simulink model "IEEE30_case"  (R2024b)
settings: Solver=FixedStepAuto  StartTime=0  StopTime=5  FixedStep=1e-7  RelTol=1e-3
values from neighbouring files (symbols this model uses):
  GFL_DFIG_7_C_bus = 0.08    [IEEE30_case_parameters.m]
  GFL_DFIG_7_D_mutual = 2.500000e+3    (= 2500)    [IEEE30_case_parameters.m]
  GFL_DFIG_7_f0 = 60    [IEEE30_case_parameters.m]
  GFL_DFIG_7_gPLLi = 3200    [IEEE30_case_parameters.m]
  GFL_DFIG_7_gPLLp = 650    [IEEE30_case_parameters.m]
  GFL_DFIG_7_H_WT = 0.4    [IEEE30_case_parameters.m]
  GFL_DFIG_7_Hg = 0.8    [IEEE30_case_parameters.m]
  GFL_DFIG_7_Igq_ref = 0    [IEEE30_case_parameters.m]
  GFL_DFIG_7_Ird_ref = 704.45696    [IEEE30_case_parameters.m]
  GFL_DFIG_7_KI_V = -300000    [IEEE30_case_parameters.m]
  GFL_DFIG_7_KP_V = -1000    [IEEE30_case_parameters.m]
  GFL_DFIG_7_Ksh = 1.254300e+4    (= 12543)    [IEEE30_case_parameters.m]
  GFL_DFIG_7_Lg = 0.000483    [IEEE30_case_parameters.m]
  GFL_DFIG_7_Lm_pu = 4    [IEEE30_case_parameters.m]
  GFL_DFIG_7_N = 100    [IEEE30_case_parameters.m]
  GFL_DFIG_7_p = 2    [IEEE30_case_parameters.m]
  GFL_DFIG_7_Pitch = 0    [IEEE30_case_parameters.m]
  GFL_DFIG_7_R = 44    [IEEE30_case_parameters.m]
  GFL_DFIG_7_Rg = 2.000000e-5    (= 2e-05)    [IEEE30_case_parameters.m]
  GFL_DFIG_7_rho = 1.225    [IEEE30_case_parameters.m]
  GFL_DFIG_7_rPLLi = 4500    [IEEE30_case_parameters.m]
  GFL_DFIG_7_rPLLp = 620    [IEEE30_case_parameters.m]
  GFL_DFIG_7_Rs_pu = 0.011    [IEEE30_case_parameters.m]
  GFL_DFIG_7_Sbase = 2.000000e+6    (= 2000000)    [IEEE30_case_parameters.m]
  GFL_DFIG_7_ugq_ref = 0    [IEEE30_case_parameters.m]
  GFL_DFIG_7_usd_ref = 0    [IEEE30_case_parameters.m]
  GFL_DFIG_7_Vbase = 690    [IEEE30_case_parameters.m]
  GFL_DFIG_7_Vdc_ref = 1200    [IEEE30_case_parameters.m]
  GFL_DFIG_7_wind = 12    [IEEE30_case_parameters.m]
  GFL_DFIG_7_wm_ref = 518.184209    [IEEE30_case_parameters.m]
  SG_D_13_D = 0.01056    [IEEE30_case_parameters.m]
  SG_D_13_EnableSaturation = 0    [IEEE30_case_parameters.m]
  SG_D_13_f0 = 60    [IEEE30_case_parameters.m]
  SG_D_13_H = 7.5    [IEEE30_case_parameters.m]
  SG_D_13_K_A = 20    [IEEE30_case_parameters.m]
  SG_D_13_K_E = 1.000000e+1    (= 10)    [IEEE30_case_parameters.m]
  SG_D_13_K_F = 2.363    [IEEE30_case_parameters.m]
  SG_D_13_K_s = 0.5    [IEEE30_case_parameters.m]
  SG_D_13_R_a = 0.001088    [IEEE30_case_parameters.m]
  SG_D_13_S_A = 1    [IEEE30_case_parameters.m]
  SG_D_13_S_B = 0.103    [IEEE30_case_parameters.m]
  SG_D_13_S_N = 10.659857    [IEEE30_case_parameters.m]
  SG_D_13_SpeedPara = 200    [IEEE30_case_parameters.m]
  SG_D_13_T_0 = 0.370163    [IEEE30_case_parameters.m]
  SG_D_13_T_1 = 0.3    [IEEE30_case_parameters.m]
  SG_D_13_T_2 = 0.05    [IEEE30_case_parameters.m]
  SG_D_13_T_3 = 0.02    [IEEE30_case_parameters.m]
  SG_D_13_T_4 = 0.005    [IEEE30_case_parameters.m]
  SG_D_13_T_A = 0.02    [IEEE30_case_parameters.m]
  SG_D_13_T_dd = 8.000000e+0    (= 8)    [IEEE30_case_parameters.m]
  SG_D_13_T_ddd = 0.04    [IEEE30_case_parameters.m]
  SG_D_13_T_E = 0.314    [IEEE30_case_parameters.m]
  SG_D_13_T_F = 0.35    [IEEE30_case_parameters.m]
  SG_D_13_T_qd = 0.8    [IEEE30_case_parameters.m]
  SG_D_13_T_qdd = 0.02    [IEEE30_case_parameters.m]
  SG_D_13_T_speed = 0.1    [IEEE30_case_parameters.m]
  SG_D_13_T_w = 0.5    [IEEE30_case_parameters.m]
  SG_D_13_V_ref = 1.696619    [IEEE30_case_parameters.m]
  SG_D_13_w_ref = 376.991118    [IEEE30_case_parameters.m]
  SG_D_13_x_d = 1.9    [IEEE30_case_parameters.m]
  SG_D_13_x_dd = 0.302    [IEEE30_case_parameters.m]
  SG_D_13_x_ddd = 0.204    [IEEE30_case_parameters.m]
  SG_D_13_x_l = 0.05    [IEEE30_case_parameters.m]
  SG_D_13_x_q = 1.3    [IEEE30_case_parameters.m]
  SG_D_13_x_qd = 0.5    [IEEE30_case_parameters.m]
  SG_D_13_x_qdd = 0.3    [IEEE30_case_parameters.m]
  SG_D_1_D = 0.01056    [IEEE30_case_parameters.m]
  SG_D_1_EnableSaturation = 0    [IEEE30_case_parameters.m]
  SG_D_1_f0 = 60    [IEEE30_case_parameters.m]
  SG_D_1_H = 7.5    [IEEE30_case_parameters.m]
  SG_D_1_K_A = 20    [IEEE30_case_parameters.m]
  SG_D_1_K_E = 1.000000e+1    (= 10)    [IEEE30_case_parameters.m]
  SG_D_1_K_F = 2.363    [IEEE30_case_parameters.m]
  SG_D_1_K_s = 0.5    [IEEE30_case_parameters.m]
  SG_D_1_R_a = 0.001088    [IEEE30_case_parameters.m]
  SG_D_1_S_A = 1    [IEEE30_case_parameters.m]
  SG_D_1_S_B = 0.103    [IEEE30_case_parameters.m]
  SG_D_1_S_N = 10.659857    [IEEE30_case_parameters.m]
  SG_D_1_SpeedPara = 200    [IEEE30_case_parameters.m]
  SG_D_1_T_0 = 0.259812    [IEEE30_case_parameters.m]
  SG_D_1_T_1 = 0.3    [IEEE30_case_parameters.m]
  SG_D_1_T_2 = 0.05    [IEEE30_case_parameters.m]
  SG_D_1_T_3 = 0.02    [IEEE30_case_parameters.m]
  SG_D_1_T_4 = 0.005    [IEEE30_case_parameters.m]
  SG_D_1_T_A = 0.02    [IEEE30_case_parameters.m]
  SG_D_1_T_dd = 8.000000e+0    (= 8)    [IEEE30_case_parameters.m]
  SG_D_1_T_ddd = 0.04    [IEEE30_case_parameters.m]
  SG_D_1_T_E = 0.314    [IEEE30_case_parameters.m]
  SG_D_1_T_F = 0.35    [IEEE30_case_parameters.m]
  SG_D_1_T_qd = 0.8    [IEEE30_case_parameters.m]
  SG_D_1_T_qdd = 0.02    [IEEE30_case_parameters.m]
  SG_D_1_T_speed = 0.1    [IEEE30_case_parameters.m]
  SG_D_1_T_w = 0.5    [IEEE30_case_parameters.m]
  SG_D_1_V_ref = 1.544107    [IEEE30_case_parameters.m]
  SG_D_1_w_ref = 376.991118    [IEEE30_case_parameters.m]
  SG_D_1_x_d = 1.9    [IEEE30_case_parameters.m]
  SG_D_1_x_dd = 0.302    [IEEE30_case_parameters.m]
  SG_D_1_x_ddd = 0.204    [IEEE30_case_parameters.m]
  SG_D_1_x_l = 0.05    [IEEE30_case_parameters.m]
  SG_D_1_x_q = 1.3    [IEEE30_case_parameters.m]
  SG_D_1_x_qd = 0.5    [IEEE30_case_parameters.m]
  SG_D_1_x_qdd = 0.3    [IEEE30_case_parameters.m]
  SG_D_22_D = 0.01056    [IEEE30_case_parameters.m]
  SG_D_22_EnableSaturation = 0    [IEEE30_case_parameters.m]
  SG_D_22_f0 = 60    [IEEE30_case_parameters.m]
  SG_D_22_H = 7.5    [IEEE30_case_parameters.m]
  SG_D_22_K_A = 20    [IEEE30_case_parameters.m]
  SG_D_22_K_E = 1.000000e+1    (= 10)    [IEEE30_case_parameters.m]
  SG_D_22_K_F = 2.363    [IEEE30_case_parameters.m]
  SG_D_22_K_s = 0.5    [IEEE30_case_parameters.m]
  SG_D_22_R_a = 0.001088    [IEEE30_case_parameters.m]
  SG_D_22_S_A = 1    [IEEE30_case_parameters.m]
  SG_D_22_S_B = 0.103    [IEEE30_case_parameters.m]
  SG_D_22_S_N = 10.659857    [IEEE30_case_parameters.m]
  SG_D_22_SpeedPara = 200    [IEEE30_case_parameters.m]
  SG_D_22_T_0 = 0.216121    [IEEE30_case_parameters.m]
  SG_D_22_T_1 = 0.3    [IEEE30_case_parameters.m]
  SG_D_22_T_2 = 0.05    [IEEE30_case_parameters.m]
  SG_D_22_T_3 = 0.02    [IEEE30_case_parameters.m]
  SG_D_22_T_4 = 0.005    [IEEE30_case_parameters.m]
  ... (+126 more)
(part 19 of 27)

== system IEEE30_case/SG_D_13/d_psi_q_SG_D_13_block ==
  note: d_psi_q_SG_D_13 in IEEE30_case
      | $2\,\pi \,f_{0}\,\left(v_{d,\mathrm{SG},D,13}\,\cos\left(\theta _{\mathrm{SG},D,13}\right)+v_{q,\mathrm{SG},D,13}\,\sin\left(\theta _{\mathrm{SG},D,13}\right)-\frac{R_{a}\,\left(\psi _{q,\mathrm{SG},D,13}+\frac{\psi _{\mathrm{gq},\mathrm{SG},D,13}\,\left(x_{l}-x_{\mathrm{qdd}}\right)}{x_{l}-x_{\mathrm{qd}}}+\frac{\psi _{\mathrm{kq},\mathrm{SG},D,13}\,\left(x_{\mathrm{qd}}-x_{\mathrm{qdd}}\right)}{x_{l}-x_{\mathrm{qd}}}\right)}{x_{\mathrm{qdd}}}-\frac{\psi _{d,\mathrm{SG},D,13}\,w_{\mathrm{SG},D,13}}{2\,f_{0}\,\pi }\right)$
      | Automatically generated on 2025-11-01 18:34:46 .
  State_psi_gq_SG_D_13_b9e70 : Inport
  State_psi_kq_SG_D_13_777e8 : Inport  Port=2
  State_psi_q_SG_D_13_352e5 : Inport  Port=3
  Input_v_d_SG_D_13_60103 : Inport  Port=4
  State_theta_SG_D_13_d73b7 : Inport  Port=5
  Input_v_q_SG_D_13_89396 : Inport  Port=6
  State_theta_SG_D_13_d24c4 : Inport  Port=7
  State_psi_d_SG_D_13_acca0 : Inport  Port=8
  State_w_SG_D_13_af3fa : Inport  Port=9
  Add_212ec : Sum
  Add_30131 : Sum
  Add_3345e : Sum
  Add_60563 : Sum
  Add_71f1c : Sum
  Constant_-1_23601 : Constant  Value=-1
  Constant_-1_802f8 : Constant  Value=-1
  Constant_-1_a74eb : Constant  Value=-1
  Constant_-2.0_d214a : Constant  Value=-2.0
  Constant_2.0_b6abe : Constant  Value=2.0
  Constant_R_a_2cc2b : Constant  Value=R_a
  Constant_f0_87ec9 : Constant  Value=f0
  Constant_f0_e30ed : Constant  Value=f0
  Constant_pi_494f1 : Constant  Value=pi
  Constant_pi_861ee : Constant  Value=pi
  Constant_x_l_134aa : Constant  Value=x_l
  Constant_x_l_cdd9f : Constant  Value=x_l
  Constant_x_l_e4e7e : Constant  Value=x_l
  Constant_x_qd_c3898 : Constant  Value=x_qd
  Constant_x_qd_e989e : Constant  Value=x_qd
  Constant_x_qd_f4ba2 : Constant  Value=x_qd
  Constant_x_qdd_25541 : Constant  Value=x_qdd
  Constant_x_qdd_713f8 : Constant  Value=x_qdd
  Constant_x_qdd_d4846 : Constant  Value=x_qdd
  Divide_26cb3 : Product  Inputs=*/
  Divide_92868 : Product  Inputs=*/
  Divide_950ba : Product  Inputs=*/
  Divide_db475 : Product  Inputs=*/
  MathFunc_cos_7503c : Trigonometry  Operator=cos
  MathFunc_sin_a8361 : Trigonometry
  Product_06178 : Product
  Product_316b1 : Product
  Product_3ac25 : Product
  Product_3c410 : Product
  Product_432cf : Product
  Product_5efb9 : Product
  Product_7509b : Product
  Product_9806d : Product
  Product_a5768 : Product
  Product_b8d96 : Product
  Product_ba2c3 : Product
  Product_bcc7a : Product
  Product_c3e4c : Product
  Product_de780 : Product
  Subtract_222ea : Sum  Inputs=+-
  Subtract_2db43 : Sum  Inputs=+-
  Subtract_b2b6c : Sum  Inputs=+-
  Subtract_cd486 : Sum  Inputs=+-
  Blockout_d_psi_q_SG_D_13_271e8 : Outport
  wires:
  Constant_f0_87ec9/1 -> Product_b8d96/2
  Constant_x_l_cdd9f/1 -> Product_316b1/2
  Constant_-1_802f8/1 -> Product_5efb9/1
  Product_5efb9/1 -> Add_212ec/1
  Subtract_222ea/1 -> Subtract_cd486/1
  Constant_x_l_e4e7e/1 -> Product_5efb9/2
  Subtract_b2b6c/1 -> Product_ba2c3/2
  Constant_x_qd_c3898/1 -> Subtract_b2b6c/1
  Constant_x_qdd_25541/1 -> Add_212ec/2
  Add_60563/1 -> Product_a5768/2
  Product_316b1/1 -> Add_71f1c/1
  Constant_-1_23601/1 -> Product_316b1/1
  Constant_-2.0_d214a/1 -> Product_432cf/1
  Constant_x_qdd_713f8/1 -> Subtract_b2b6c/2
  Constant_pi_861ee/1 -> Product_de780/2
  Product_a5768/1 -> Divide_92868/1
  Product_9806d/1 -> Add_30131/1
  Constant_-1_a74eb/1 -> Product_9806d/1
  Constant_x_l_134aa/1 -> Product_9806d/2
  Subtract_cd486/1 -> Add_3345e/1
  Product_c3e4c/1 -> Divide_950ba/1
  Constant_x_qd_e989e/1 -> Add_71f1c/2
  State_psi_gq_SG_D_13_b9e70/1 -> Product_c3e4c/1
  Add_212ec/1 -> Product_c3e4c/2
  Product_ba2c3/1 -> Divide_26cb3/1
  State_psi_kq_SG_D_13_777e8/1 -> Product_ba2c3/1
  Product_bcc7a/1 -> Divide_db475/2
  Constant_x_qd_f4ba2/1 -> Add_30131/2
  Add_71f1c/1 -> Divide_950ba/2
  Product_b8d96/1 -> Product_3ac25/1
  Add_30131/1 -> Divide_26cb3/2
  Divide_950ba/1 -> Subtract_2db43/1
  Subtract_2db43/1 -> Add_60563/1
  Divide_26cb3/1 -> Subtract_2db43/2
  State_psi_q_SG_D_13_352e5/1 -> Add_60563/2
  Product_3c410/1 -> Subtract_cd486/2
  Constant_R_a_2cc2b/1 -> Product_a5768/1
  State_theta_SG_D_13_d73b7/1 -> MathFunc_cos_7503c/1
  Constant_x_qdd_d4846/1 -> Divide_92868/2
  Product_7509b/1 -> Subtract_222ea/2
  Input_v_d_SG_D_13_60103/1 -> Product_7509b/1
  MathFunc_cos_7503c/1 -> Product_7509b/2
  Constant_f0_e30ed/1 -> Product_bcc7a/2
  MathFunc_sin_a8361/1 -> Product_3c410/2
  State_theta_SG_D_13_d24c4/1 -> MathFunc_sin_a8361/1
  Product_de780/1 -> Product_bcc7a/1
  Constant_2.0_b6abe/1 -> Product_de780/1
  Divide_92868/1 -> Subtract_222ea/1
  Input_v_q_SG_D_13_89396/1 -> Product_3c410/1
  Product_06178/1 -> Divide_db475/1
  State_psi_d_SG_D_13_acca0/1 -> Product_06178/1
  State_w_SG_D_13_af3fa/1 -> Product_06178/2
  Constant_pi_494f1/1 -> Product_432cf/2
  Divide_db475/1 -> Add_3345e/2
  Product_432cf/1 -> Product_b8d96/1
  Add_3345e/1 -> Product_3ac25/2
  Product_3ac25/1 -> Blockout_d_psi_q_SG_D_13_271e8/1

== system IEEE30_case/SG_D_13/d_theta_SG_D_13_block ==
  note: d_theta_SG_D_13 in IEEE30_case
      | $w_{\mathrm{SG},D,13}-2\,\pi \,f_{0}$
      | Automatically generated on 2025-11-01 18:35:09 .
  State_w_SG_D_13_8eb78 : Inport
  Add_5b0be : Sum
  Constant_-2.0_19a96 : Constant  Value=-2.0
  Constant_f0_3b1b7 : Constant  Value=f0
  Constant_pi_8ca32 : Constant  Value=pi
  Product_6dbd8 : Product
  Product_d020b : Product
  Blockout_d_theta_SG_D_13_8df5a : Outport
  wires:
  Constant_-2.0_19a96/1 -> Product_d020b/1
  Constant_pi_8ca32/1 -> Product_d020b/2
  Product_d020b/1 -> Product_6dbd8/1
  Constant_f0_3b1b7/1 -> Product_6dbd8/2
  Product_6dbd8/1 -> Add_5b0be/1
  State_w_SG_D_13_8eb78/1 -> Add_5b0be/2
  Add_5b0be/1 -> Blockout_d_theta_SG_D_13_8df5a/1

== system IEEE30_case/SG_D_13/d_w_SG_D_13_block ==
  note: d_w_SG_D_13 in IEEE30_case
      | $\frac{2\,\pi \,T_{m,\mathrm{SG},D,13}\,f_{0}-D\,\left(w_{\mathrm{SG},D,13}-2\,\pi \,f_{0}\right)+2\,\pi \,f_{0}\,\left(\frac{\psi _{d,\mathrm{SG},D,13}\,\left(\psi _{q,\mathrm{SG},D,13}+\frac{\psi _{\mathrm{gq},\mathrm{SG},D,13}\,\left(x_{l}-x_{\mathrm{qdd}}\right)}{x_{l}-x_{\mathrm{qd}}}+\frac{\psi _{\mathrm{kq},\mathrm{SG},D,13}\,\left(x_{\mathrm{qd}}-x_{\mathrm{qdd}}\right)}{x_{l}-x_{\mathrm{qd}}}\right)}{x_{\mathrm{qdd}}}+\frac{\psi _{q,\mathrm{SG},D,13}\,\left(\frac{\psi _{\mathrm{1d},\mathrm{SG},D,13}\,\left(x_{\mathrm{dd}}-x_{\mathrm{ddd}}\right)}{x_{\mathrm{dd}}-x_{l}}-\psi _{d,\mathrm{SG},D,13}+\frac{\psi _{\mathrm{fd},\mathrm{SG},D,13}\,\left(x_{\mathrm{ddd}}-x_{l}\right)}{x_{\mathrm{dd}}-x_{l}}\right)}{x_{\mathrm{ddd}}}\right)}{2\,H}$
      | Automatically generated on 2025-11-01 18:35:08 .
  State_w_SG_D_13_19ab7 : Inport
  State_T_m_SG_D_13_4085f : Inport  Port=2
  State_psi_d_SG_D_13_11de5 : Inport  Port=3
  State_psi_gq_SG_D_13_70bd9 : Inport  Port=4
  State_psi_kq_SG_D_13_63ece : Inport  Port=5
  State_psi_q_SG_D_13_5c293 : Inport  Port=6
  State_psi_q_SG_D_13_4a816 : Inport  Port=7
  State_psi_1d_SG_D_13_7983e : Inport  Port=8
  State_psi_d_SG_D_13_5219f : Inport  Port=9
  State_psi_fd_SG_D_13_7ff7c : Inport  Port=10
  Add_13550 : Sum
  Add_44288 : Sum
  Add_541be : Sum
  Add_55ae8 : Sum
  Add_79725 : Sum
  Add_cedf2 : Sum
  Add_e732f : Sum
  Add_f4421 : Sum
  Constant_-1_301db : Constant  Value=-1
  Constant_-1_73986 : Constant  Value=-1
  Constant_-1_b6954 : Constant  Value=-1
  Constant_-1_c944e : Constant  Value=-1
  Constant_-1_feeb7 : Constant  Value=-1
  Constant_-1_fef2a : Constant  Value=-1
  Constant_-2.0_0ea0b : Constant  Value=-2.0
  Constant_2.0_248bb : Constant  Value=2.0
  Constant_2.0_71a88 : Constant  Value=2.0
  Constant_2.0_c924b : Constant  Value=2.0
  Constant_D_edeba : Constant  Value=D
  Constant_H_fa43f : Constant  Value=H
  Constant_f0_5fd3b : Constant  Value=f0
  Constant_f0_77476 : Constant  Value=f0
  Constant_f0_7887e : Constant  Value=f0
  Constant_pi_3bfc5 : Constant  Value=pi
  Constant_pi_41a94 : Constant  Value=pi
  Constant_pi_443e6 : Constant  Value=pi
  Constant_x_dd_1b9c9 : Constant  Value=x_dd
  Constant_x_dd_47ce8 : Constant  Value=x_dd
  Constant_x_dd_c5806 : Constant  Value=x_dd
  Constant_x_ddd_50ef7 : Constant  Value=x_ddd
  Constant_x_ddd_9135a : Constant  Value=x_ddd
  Constant_x_ddd_eed82 : Constant  Value=x_ddd
  Constant_x_l_0d788 : Constant  Value=x_l
  Constant_x_l_44bb8 : Constant  Value=x_l
  Constant_x_l_4908c : Constant  Value=x_l
  Constant_x_l_5bd13 : Constant  Value=x_l
  Constant_x_l_6d3ab : Constant  Value=x_l
  Constant_x_l_8c27d : Constant  Value=x_l
  Constant_x_qd_0dc72 : Constant  Value=x_qd
  Constant_x_qd_34db0 : Constant  Value=x_qd
  Constant_x_qd_dbd1d : Constant  Value=x_qd
  Constant_x_qdd_780b2 : Constant  Value=x_qdd
  Constant_x_qdd_cb49a : Constant  Value=x_qdd
  Constant_x_qdd_edc06 : Constant  Value=x_qdd
  Divide_0c8e5 : Product  Inputs=*/
  Divide_1fc9d : Product  Inputs=*/
  Divide_2629b : Product  Inputs=*/
  Divide_79611 : Product  Inputs=*/
  Divide_ba4e7 : Product  Inputs=*/
  Divide_d65ea : Product  Inputs=*/
  Divide_faefc : Product  Inputs=*/
  Product_0b906 : Product
  Product_1de22 : Product
  Product_29e89 : Product
  Product_316ea : Product
  Product_45e42 : Product
  Product_4a016 : Product
  Product_50369 : Product
  Product_6e93f : Product
  Product_7fe14 : Product
  Product_8575f : Product
  Product_8b6f1 : Product
  Product_9652d : Product
  Product_a32aa : Product
  Product_b5314 : Product
  Product_b5db7 : Product
  Product_bba2e : Product
  Product_bd01c : Product
  Product_c33c5 : Product
  Product_dec30 : Product
  Product_e26d7 : Product
  Product_eaa2d : Product
  Product_ed00b : Product
  Subtract_20a7a : Sum  Inputs=+-
  Subtract_5cf3c : Sum  Inputs=+-
  Subtract_6ad0f : Sum  Inputs=+-
  Subtract_74c58 : Sum  Inputs=+-
  Subtract_811b3 : Sum  Inputs=+-
  Subtract_9d08d : Sum  Inputs=+-
  Subtract_de186 : Sum  Inputs=+-
  Subtract_e8d44 : Sum  Inputs=+-
  Blockout_d_w_SG_D_13_b8f6b : Outport
  wires:
  Constant_-1_fef2a/1 -> Product_eaa2d/1
  Constant_x_l_6d3ab/1 -> Product_eaa2d/2
  Product_1de22/1 -> Add_cedf2/1
  Constant_x_l_5bd13/1 -> Product_b5314/2
  Product_eaa2d/1 -> Add_44288/1
  Constant_2.0_248bb/1 -> Product_29e89/1
  Constant_x_qdd_edc06/1 -> Add_44288/2
  Constant_-1_feeb7/1 -> Product_b5314/1
  Product_9652d/1 -> Product_dec30/1
  Constant_x_qd_dbd1d/1 -> Add_13550/2
  Constant_x_qd_34db0/1 -> Subtract_20a7a/1
  Constant_x_qdd_cb49a/1 -> Subtract_20a7a/2
  Constant_-1_c944e/1 -> Product_1de22/1
  Constant_x_l_8c27d/1 -> Product_1de22/2
  Product_ed00b/1 -> Product_8575f/1
  Constant_-1_301db/1 -> Product_ed00b/1
  State_psi_1d_SG_D_13_7983e/1 -> Product_ed00b/2
  Subtract_de186/1 -> Product_8575f/2
  Constant_x_dd_1b9c9/1 -> Subtract_de186/1
  Constant_x_ddd_50ef7/1 -> Subtract_de186/2
  State_psi_d_SG_D_13_11de5/1 -> Product_bba2e/2
  State_psi_gq_SG_D_13_70bd9/1 -> Product_b5db7/1
  Constant_H_fa43f/1 -> Product_29e89/2
  Add_44288/1 -> Product_b5db7/2
  Product_b5314/1 -> Add_13550/1
  State_psi_kq_SG_D_13_63ece/1 -> Product_8b6f1/1
  Subtract_20a7a/1 -> Product_8b6f1/2
  Add_13550/1 -> Divide_0c8e5/2
  Add_e732f/1 -> Product_dec30/2
  Constant_x_qd_0dc72/1 -> Add_cedf2/2
  Subtract_e8d44/1 -> Divide_1fc9d/2
  Constant_x_dd_47ce8/1 -> Subtract_e8d44/1
  State_w_SG_D_13_19ab7/1 -> Add_e732f/2
  Product_0b906/1 -> Product_316ea/1
  Constant_x_dd_c5806/1 -> Subtract_74c58/1
  Constant_x_l_0d788/1 -> Subtract_e8d44/2
  Constant_pi_3bfc5/1 -> Product_45e42/2
  Constant_x_ddd_eed82/1 -> Subtract_9d08d/1
  Constant_2.0_c924b/1 -> Product_45e42/1
  State_psi_fd_SG_D_13_7ff7c/1 -> Product_c33c5/1
  Constant_x_l_4908c/1 -> Subtract_9d08d/2
  Product_b5db7/1 -> Divide_0c8e5/1
  Product_8b6f1/1 -> Divide_d65ea/1
  Add_cedf2/1 -> Divide_d65ea/2
  Product_8575f/1 -> Divide_1fc9d/1
  Subtract_9d08d/1 -> Product_c33c5/2
  Constant_x_l_44bb8/1 -> Subtract_74c58/2
  Divide_0c8e5/1 -> Subtract_811b3/1
  Divide_d65ea/1 -> Subtract_811b3/2
  Divide_1fc9d/1 -> Add_55ae8/1
  State_psi_d_SG_D_13_5219f/1 -> Add_55ae8/2
  Product_c33c5/1 -> Divide_79611/1
  Subtract_74c58/1 -> Divide_79611/2
  Constant_-2.0_0ea0b/1 -> Product_50369/1
  Constant_pi_41a94/1 -> Product_50369/2
  Constant_-1_73986/1 -> Product_bba2e/1
  Subtract_811b3/1 -> Add_f4421/1
  Product_bd01c/1 -> Add_e732f/1
  State_psi_q_SG_D_13_5c293/1 -> Add_f4421/2
  Add_55ae8/1 -> Subtract_5cf3c/1
  Divide_79611/1 -> Subtract_5cf3c/2
  Product_50369/1 -> Product_bd01c/1
  Constant_f0_5fd3b/1 -> Product_bd01c/2
  Constant_-1_b6954/1 -> Product_9652d/1
  Product_bba2e/1 -> Product_4a016/1
  Add_f4421/1 -> Product_4a016/2
  State_psi_q_SG_D_13_4a816/1 -> Product_e26d7/1
  Subtract_5cf3c/1 -> Product_e26d7/2
  Constant_D_edeba/1 -> Product_9652d/2
  Product_45e42/1 -> Product_a32aa/1
  State_T_m_SG_D_13_4085f/1 -> Product_a32aa/2
  Constant_2.0_71a88/1 -> Product_6e93f/1
  Constant_pi_443e6/1 -> Product_6e93f/2
  Product_4a016/1 -> Divide_2629b/1
  Constant_x_qdd_780b2/1 -> Divide_2629b/2
  Product_e26d7/1 -> Divide_faefc/1
  Constant_x_ddd_9135a/1 -> Divide_faefc/2
  Product_a32aa/1 -> Product_7fe14/1
  Constant_f0_7887e/1 -> Product_7fe14/2
  Product_6e93f/1 -> Product_0b906/1
  Constant_f0_77476/1 -> Product_0b906/2
  Divide_2629b/1 -> Add_79725/1
  Divide_faefc/1 -> Add_79725/2
  Product_dec30/1 -> Add_541be/1
  Product_7fe14/1 -> Add_541be/2
  Add_79725/1 -> Product_316ea/2
  Add_541be/1 -> Subtract_6ad0f/1
  Product_316ea/1 -> Subtract_6ad0f/2
  Subtract_6ad0f/1 -> Divide_ba4e7/1
  Product_29e89/1 -> Divide_ba4e7/2
  Divide_ba4e7/1 -> Blockout_d_w_SG_D_13_b8f6b/1

== system IEEE30_case/SG_D_13/i_d_SG_D_13_block ==
  note: i_d_SG_D_13 in IEEE30_case
      | $\frac{\sin\left(\theta _{\mathrm{SG},D,13}\right)\,\left(\frac{\psi _{\mathrm{1d},\mathrm{SG},D,13}\,\left(x_{\mathrm{dd}}-x_{\mathrm{ddd}}\right)}{x_{\mathrm{dd}}-x_{l}}-\psi _{d,\mathrm{SG},D,13}+\frac{\psi _{\mathrm{fd},\mathrm{SG},D,13}\,\left(x_{\mathrm{ddd}}-x_{l}\right)}{x_{\mathrm{dd}}-x_{l}}\right)}{x_{\mathrm{ddd}}}-\frac{\cos\left(\theta _{\mathrm{SG},D,13}\right)\,\left(\psi _{q,\mathrm{SG},D,13}+\frac{\psi _{\mathrm{gq},\mathrm{SG},D,13}\,\left(x_{l}-x_{\mathrm{qdd}}\right)}{x_{l}-x_{\mathrm{qd}}}+\frac{\psi _{\mathrm{kq},\mathrm{SG},D,13}\,\left(x_{\mathrm{qd}}-x_{\mathrm{qdd}}\right)}{x_{l}-x_{\mathrm{qd}}}\right)}{x_{\mathrm{qdd}}}$
      | Automatically generated on 2025-11-01 18:35:29 .
  State_psi_gq_SG_D_13_121f4 : Inport
  State_psi_kq_SG_D_13_7664a : Inport  Port=2
  State_psi_q_SG_D_13_649a2 : Inport  Port=3
  State_theta_SG_D_13_1a75b : Inport  Port=4
  State_psi_1d_SG_D_13_cb17c : Inport  Port=5
  State_psi_d_SG_D_13_e9088 : Inport  Port=6
  State_psi_fd_SG_D_13_9dba0 : Inport  Port=7
  State_theta_SG_D_13_6f0a0 : Inport  Port=8
  Add_0d65a : Sum
  Add_201bb : Sum
  Add_8664e : Sum
  Add_a9e64 : Sum
  Add_fce67 : Sum
  Constant_-1_456d2 : Constant  Value=-1
  Constant_-1_46e43 : Constant  Value=-1
  Constant_-1_9970b : Constant  Value=-1
  Constant_-1_d4ce2 : Constant  Value=-1
  Constant_-1_d7eea : Constant  Value=-1
  Constant_x_dd_568b7 : Constant  Value=x_dd
  Constant_x_dd_b9b42 : Constant  Value=x_dd
  Constant_x_dd_f3f3e : Constant  Value=x_dd
  Constant_x_ddd_208b9 : Constant  Value=x_ddd
  Constant_x_ddd_4409e : Constant  Value=x_ddd
  Constant_x_ddd_6af1a : Constant  Value=x_ddd
  Constant_x_l_113f1 : Constant  Value=x_l
  Constant_x_l_1d021 : Constant  Value=x_l
  Constant_x_l_8998a : Constant  Value=x_l
  Constant_x_l_97258 : Constant  Value=x_l
  Constant_x_l_c21c1 : Constant  Value=x_l
  Constant_x_l_c559c : Constant  Value=x_l
  Constant_x_qd_00493 : Constant  Value=x_qd
  Constant_x_qd_21d9e : Constant  Value=x_qd
  Constant_x_qd_da2ed : Constant  Value=x_qd
  Constant_x_qdd_5f056 : Constant  Value=x_qdd
  Constant_x_qdd_cf6b9 : Constant  Value=x_qdd
  Constant_x_qdd_d0c9b : Constant  Value=x_qdd
  Divide_04736 : Product  Inputs=*/
  Divide_21963 : Product  Inputs=*/
  Divide_7735c : Product  Inputs=*/
  Divide_7a170 : Product  Inputs=*/
  Divide_c2433 : Product  Inputs=*/
  Divide_e94fb : Product  Inputs=*/
  MathFunc_cos_c11eb : Trigonometry  Operator=cos
  MathFunc_sin_dd9a3 : Trigonometry
  Product_1b6b8 : Product
  Product_36d30 : Product
  Product_38cb1 : Product
  Product_3919d : Product
  Product_60700 : Product
  Product_8dbd4 : Product
  Product_a4101 : Product
  Product_aa04e : Product
  Product_b7237 : Product
  Product_e18b6 : Product
  Product_ef241 : Product
  Subtract_{30933,67967,73410,74097} (4 alike) : Sum  Inputs=+-
  Subtract_574f5 : Sum  Inputs=+-
  Subtract_5ba01 : Sum  Inputs=+-
  Subtract_8df3f : Sum  Inputs=+-
  Subtract_b18cc : Sum  Inputs=+-
  Blockout_i_d_SG_D_13_47119 : Outport
  wires:
  Constant_x_ddd_6af1a/1 -> Subtract_5ba01/1
  Product_60700/1 -> Add_0d65a/1
  Constant_-1_d7eea/1 -> Product_60700/1
  Constant_x_qdd_d0c9b/1 -> Add_a9e64/2
  Divide_21963/1 -> Add_fce67/1
  Constant_-1_d4ce2/1 -> Product_aa04e/1
  Product_aa04e/1 -> Add_a9e64/1
  Subtract_30933/1 -> Product_36d30/2
  Add_0d65a/1 -> Divide_c2433/2
  Constant_x_dd_568b7/1 -> Subtract_30933/1
  Constant_x_l_c21c1/1 -> Product_aa04e/2
  Product_38cb1/1 -> Add_201bb/1
  Constant_-1_9970b/1 -> Product_38cb1/1
  Subtract_74097/1 -> Product_8dbd4/2
  Constant_x_l_97258/1 -> Product_38cb1/2
  Constant_x_qd_00493/1 -> Subtract_74097/1
  Product_36d30/1 -> Divide_21963/1
  Constant_x_qdd_5f056/1 -> Subtract_74097/2
  Constant_x_l_8998a/1 -> Product_60700/2
  State_theta_SG_D_13_6f0a0/1 -> MathFunc_sin_dd9a3/1
  State_psi_gq_SG_D_13_121f4/1 -> Product_b7237/1
  Add_a9e64/1 -> Product_b7237/2
  Subtract_5ba01/1 -> Product_a4101/2
  Divide_c2433/1 -> Subtract_73410/2
  Constant_x_qd_da2ed/1 -> Add_201bb/2
  Product_8dbd4/1 -> Divide_c2433/1
  State_psi_kq_SG_D_13_7664a/1 -> Product_8dbd4/1
  Constant_x_qd_21d9e/1 -> Add_0d65a/2
  Product_e18b6/1 -> Product_36d30/1
  Constant_-1_46e43/1 -> Product_e18b6/1
  Product_a4101/1 -> Divide_7a170/1
  State_psi_1d_SG_D_13_cb17c/1 -> Product_e18b6/2
  MathFunc_cos_c11eb/1 -> Product_3919d/2
  Constant_x_ddd_208b9/1 -> Subtract_30933/2
  Product_b7237/1 -> Divide_e94fb/1
  Divide_7a170/1 -> Subtract_b18cc/2
  Add_201bb/1 -> Divide_e94fb/2
  Subtract_574f5/1 -> Divide_21963/2
  Constant_x_dd_b9b42/1 -> Subtract_574f5/1
  Constant_x_l_c559c/1 -> Subtract_574f5/2
  Subtract_b18cc/1 -> Product_ef241/1
  Constant_x_l_113f1/1 -> Subtract_5ba01/2
  Divide_e94fb/1 -> Subtract_73410/1
  State_psi_fd_SG_D_13_9dba0/1 -> Product_a4101/1
  Constant_x_dd_f3f3e/1 -> Subtract_67967/1
  Product_ef241/1 -> Divide_7735c/1
  Constant_x_l_1d021/1 -> Subtract_67967/2
  Subtract_73410/1 -> Add_8664e/1
  State_psi_q_SG_D_13_649a2/1 -> Add_8664e/2
  State_psi_d_SG_D_13_e9088/1 -> Add_fce67/2
  Subtract_67967/1 -> Divide_7a170/2
  Constant_-1_456d2/1 -> Product_1b6b8/1
  Add_8664e/1 -> Product_1b6b8/2
  State_theta_SG_D_13_1a75b/1 -> MathFunc_cos_c11eb/1
  Add_fce67/1 -> Subtract_b18cc/1
  Product_1b6b8/1 -> Product_3919d/1
  MathFunc_sin_dd9a3/1 -> Product_ef241/2
  Product_3919d/1 -> Divide_04736/1
  Constant_x_qdd_cf6b9/1 -> Divide_04736/2
  Constant_x_ddd_4409e/1 -> Divide_7735c/2
  Divide_7735c/1 -> Subtract_8df3f/2
  Divide_04736/1 -> Subtract_8df3f/1
  Subtract_8df3f/1 -> Blockout_i_d_SG_D_13_47119/1

== system IEEE30_case/SG_D_13/i_q_SG_D_13_block ==
  note: i_q_SG_D_13 in IEEE30_case
      | $-\frac{\sin\left(\theta _{\mathrm{SG},D,13}\right)\,\left(\psi _{q,\mathrm{SG},D,13}+\frac{\psi _{\mathrm{gq},\mathrm{SG},D,13}\,\left(x_{l}-x_{\mathrm{qdd}}\right)}{x_{l}-x_{\mathrm{qd}}}+\frac{\psi _{\mathrm{kq},\mathrm{SG},D,13}\,\left(x_{\mathrm{qd}}-x_{\mathrm{qdd}}\right)}{x_{l}-x_{\mathrm{qd}}}\right)}{x_{\mathrm{qdd}}}-\frac{\cos\left(\theta _{\mathrm{SG},D,13}\right)\,\left(\frac{\psi _{\mathrm{1d},\mathrm{SG},D,13}\,\left(x_{\mathrm{dd}}-x_{\mathrm{ddd}}\right)}{x_{\mathrm{dd}}-x_{l}}-\psi _{d,\mathrm{SG},D,13}+\frac{\psi _{\mathrm{fd},\mathrm{SG},D,13}\,\left(x_{\mathrm{ddd}}-x_{l}\right)}{x_{\mathrm{dd}}-x_{l}}\right)}{x_{\mathrm{ddd}}}$
      | Automatically generated on 2025-11-01 18:35:33 .
  State_psi_gq_SG_D_13_381c7 : Inport
  State_psi_kq_SG_D_13_c3f80 : Inport  Port=2
  State_psi_q_SG_D_13_b9242 : Inport  Port=3
  State_theta_SG_D_13_aa038 : Inport  Port=4
  State_psi_1d_SG_D_13_71e2a : Inport  Port=5
  State_psi_d_SG_D_13_cb45e : Inport  Port=6
  State_psi_fd_SG_D_13_eeae7 : Inport  Port=7
  State_theta_SG_D_13_016c8 : Inport  Port=8
  Add_0e645 : Sum
  Add_203ac : Sum
  Add_5005d : Sum
  Add_651e3 : Sum
  Add_b2a49 : Sum
  Add_fea6c : Sum
  Constant_-1_623f8 : Constant  Value=-1
  Constant_-1_69640 : Constant  Value=-1
  Constant_-1_8ebd9 : Constant  Value=-1
  Constant_-1_a02b7 : Constant  Value=-1
  Constant_-1_b1be2 : Constant  Value=-1
  Constant_x_dd_c5b13 : Constant  Value=x_dd
  Constant_x_dd_d7695 : Constant  Value=x_dd
  Constant_x_dd_f369d : Constant  Value=x_dd
  Constant_x_ddd_003ea : Constant  Value=x_ddd
  Constant_x_ddd_106e3 : Constant  Value=x_ddd
  Constant_x_ddd_271f0 : Constant  Value=x_ddd
  Constant_x_l_10a7a : Constant  Value=x_l
  Constant_x_l_20ef1 : Constant  Value=x_l
  Constant_x_l_55f41 : Constant  Value=x_l
  Constant_x_l_a0224 : Constant  Value=x_l
  Constant_x_l_b43d3 : Constant  Value=x_l
  Constant_x_l_eb5ae : Constant  Value=x_l
  Constant_x_qd_2cb0b : Constant  Value=x_qd
  Constant_x_qd_54ffc : Constant  Value=x_qd
  Constant_x_qd_c554f : Constant  Value=x_qd
  Constant_x_qdd_049f5 : Constant  Value=x_qdd
  Constant_x_qdd_31657 : Constant  Value=x_qdd
  Constant_x_qdd_9bbba : Constant  Value=x_qdd
  Divide_4bbc8 : Product  Inputs=*/
  Divide_6623b : Product  Inputs=*/
  Divide_6a102 : Product  Inputs=*/
  Divide_70f70 : Product  Inputs=*/
  Divide_bc283 : Product  Inputs=*/
  Divide_eba0c : Product  Inputs=*/
  MathFunc_cos_c135f : Trigonometry  Operator=cos
  MathFunc_sin_ffa62 : Trigonometry
  Product_2941a : Product
  Product_37b59 : Product
  Product_4ce90 : Product
  Product_50593 : Product
  Product_6067a : Product
  Product_6399d : Product
  Product_75851 : Product
  Product_93225 : Product
  Product_a4313 : Product
  Product_a7c75 : Product
  Product_c612e : Product
  Subtract_3f9d2 : Sum  Inputs=+-
  Subtract_9716f : Sum  Inputs=+-
  Subtract_a1ae8 : Sum  Inputs=+-
  Subtract_a89e6 : Sum  Inputs=+-
  Subtract_d2d5b : Sum  Inputs=+-
  Subtract_e1cfb : Sum  Inputs=+-
  Subtract_f5929 : Sum  Inputs=+-
  Blockout_i_q_SG_D_13_d5b5c : Outport
  wires:
  Product_75851/1 -> Divide_70f70/1
  Constant_x_l_55f41/1 -> Product_a7c75/2
  Product_93225/1 -> Divide_4bbc8/1
  Constant_-1_a02b7/1 -> Product_a7c75/1
  Subtract_d2d5b/1 -> Product_93225/1
  Product_a7c75/1 -> Add_651e3/1
  Constant_x_qdd_9bbba/1 -> Subtract_a89e6/2
  Constant_x_qdd_31657/1 -> Add_651e3/2
  Constant_-1_69640/1 -> Product_a4313/1
  Constant_x_dd_c5b13/1 -> Subtract_e1cfb/1
  Constant_x_l_b43d3/1 -> Product_a4313/2
  Constant_x_qd_c554f/1 -> Subtract_a89e6/1
  Constant_x_ddd_106e3/1 -> Subtract_f5929/2
  Constant_-1_623f8/1 -> Product_6399d/1
  Constant_x_dd_d7695/1 -> Subtract_f5929/1
  Constant_x_l_10a7a/1 -> Product_6399d/2
  State_psi_gq_SG_D_13_381c7/1 -> Product_50593/1
  Add_651e3/1 -> Product_50593/2
  Product_a4313/1 -> Add_5005d/1
  Constant_x_qd_2cb0b/1 -> Add_5005d/2
  Divide_6623b/1 -> Add_b2a49/1
  State_psi_kq_SG_D_13_c3f80/1 -> Product_75851/1
  Subtract_a89e6/1 -> Product_75851/2
  Constant_x_l_a0224/1 -> Subtract_a1ae8/2
  Product_6399d/1 -> Add_203ac/1
  Constant_x_qd_54ffc/1 -> Add_203ac/2
  Add_5005d/1 -> Divide_eba0c/2
  Constant_-1_b1be2/1 -> Product_c612e/1
  MathFunc_sin_ffa62/1 -> Product_37b59/2
  State_theta_SG_D_13_aa038/1 -> MathFunc_sin_ffa62/1
  State_psi_1d_SG_D_13_71e2a/1 -> Product_c612e/2
  Product_50593/1 -> Divide_eba0c/1
  Add_b2a49/1 -> Blockout_i_q_SG_D_13_d5b5c/1
  Add_203ac/1 -> Divide_70f70/2
  Product_37b59/1 -> Divide_6623b/1
  Product_c612e/1 -> Product_4ce90/1
  State_psi_q_SG_D_13_b9242/1 -> Add_fea6c/2
  Subtract_f5929/1 -> Product_4ce90/2
  Constant_x_dd_f369d/1 -> Subtract_a1ae8/1
  Constant_x_ddd_271f0/1 -> Subtract_9716f/1
  Constant_x_l_20ef1/1 -> Subtract_9716f/2
  Divide_eba0c/1 -> Subtract_3f9d2/1
  Divide_70f70/1 -> Subtract_3f9d2/2
  State_psi_d_SG_D_13_cb45e/1 -> Add_0e645/2
  Product_4ce90/1 -> Divide_6a102/1
  Subtract_a1ae8/1 -> Divide_6a102/2
  State_psi_fd_SG_D_13_eeae7/1 -> Product_6067a/1
  Subtract_9716f/1 -> Product_6067a/2
  Constant_-1_8ebd9/1 -> Product_2941a/1
  Constant_x_l_eb5ae/1 -> Subtract_e1cfb/2
  Subtract_3f9d2/1 -> Add_fea6c/1
  Divide_6a102/1 -> Add_0e645/1
  Product_6067a/1 -> Divide_bc283/1
  Subtract_e1cfb/1 -> Divide_bc283/2
  Add_fea6c/1 -> Product_2941a/2
  Product_2941a/1 -> Product_37b59/1
  Add_0e645/1 -> Subtract_d2d5b/1
  Divide_bc283/1 -> Subtract_d2d5b/2
  State_theta_SG_D_13_016c8/1 -> MathFunc_cos_c135f/1
  MathFunc_cos_c135f/1 -> Product_93225/2
  Constant_x_qdd_049f5/1 -> Divide_6623b/2
  Constant_x_ddd_003ea/1 -> Divide_4bbc8/2
  Divide_4bbc8/1 -> Add_b2a49/2

== system IEEE30_case/SG_D_13/theta_SG_D_13_out_block ==
  note: theta_SG_D_13_out in IEEE30_case
      | $\theta _{\mathrm{SG},D,13}$
      | Automatically generated on 2025-11-01 18:35:38 .
  State_theta_SG_D_13_4a098 : Inport
  Blockout_theta_SG_D_13_out_b8705 : Outport
  wires:
  State_theta_SG_D_13_4a098/1 -> Blockout_theta_SG_D_13_out_b8705/1

== system IEEE30_case/SG_D_13/w_SG_D_13_out_block ==
  note: w_SG_D_13_out in IEEE30_case
      | $w_{\mathrm{SG},D,13}$
      | Automatically generated on 2025-11-01 18:35:38 .
  State_w_SG_D_13_75d42 : Inport
  Blockout_w_SG_D_13_out_dacbe : Outport
  wires:
  State_w_SG_D_13_75d42/1 -> Blockout_w_SG_D_13_out_dacbe/1

== system IEEE30_case/SG_D_2/T_e_SG_D_2_block ==
  note: T_e_SG_D_2 in IEEE30_case
      | $-\frac{\psi _{d,\mathrm{SG},D,2}\,\left(\psi _{q,\mathrm{SG},D,2}+\frac{\psi _{\mathrm{gq},\mathrm{SG},D,2}\,\left(x_{l}-x_{\mathrm{qdd}}\right)}{x_{l}-x_{\mathrm{qd}}}+\frac{\psi _{\mathrm{kq},\mathrm{SG},D,2}\,\left(x_{\mathrm{qd}}-x_{\mathrm{qdd}}\right)}{x_{l}-x_{\mathrm{qd}}}\right)}{x_{\mathrm{qdd}}}-\frac{\psi _{q,\mathrm{SG},D,2}\,\left(\frac{\psi _{\mathrm{1d},\mathrm{SG},D,2}\,\left(x_{\mathrm{dd}}-x_{\mathrm{ddd}}\right)}{x_{\mathrm{dd}}-x_{l}}-\psi _{d,\mathrm{SG},D,2}+\frac{\psi _{\mathrm{fd},\mathrm{SG},D,2}\,\left(x_{\mathrm{ddd}}-x_{l}\right)}{x_{\mathrm{dd}}-x_{l}}\right)}{x_{\mathrm{ddd}}}$
      | Automatically generated on 2025-11-01 18:32:01 .
  State_psi_d_SG_D_2_5c155 : Inport
  State_psi_gq_SG_D_2_e2d2d : Inport  Port=2
  State_psi_kq_SG_D_2_b5b81 : Inport  Port=3
  State_psi_q_SG_D_2_2791a : Inport  Port=4
  State_psi_q_SG_D_2_b8bd3 : Inport  Port=5
  State_psi_1d_SG_D_2_ae46f : Inport  Port=6
  State_psi_d_SG_D_2_c3c7e : Inport  Port=7
  State_psi_fd_SG_D_2_fdba3 : Inport  Port=8
  Add_1b351 : Sum
  Add_1c286 : Sum
  Add_8d046 : Sum
  Add_90198 : Sum
  Add_e4b0b : Sum
  Add_e613b : Sum
  Constant_-1_0c5b4 : Constant  Value=-1
  Constant_-1_82549 : Constant  Value=-1
  Constant_-1_84d88 : Constant  Value=-1
  Constant_-1_b2676 : Constant  Value=-1
  Constant_-1_ef431 : Constant  Value=-1
  Constant_x_dd_02821 : Constant  Value=x_dd
  Constant_x_dd_0cca3 : Constant  Value=x_dd
  Constant_x_dd_59712 : Constant  Value=x_dd
  Constant_x_ddd_321b6 : Constant  Value=x_ddd
  Constant_x_ddd_94546 : Constant  Value=x_ddd
  Constant_x_ddd_b1f49 : Constant  Value=x_ddd
  Constant_x_l_34d03 : Constant  Value=x_l
  Constant_x_l_99a40 : Constant  Value=x_l
  Constant_x_l_b2fa4 : Constant  Value=x_l
  Constant_x_l_d57ae : Constant  Value=x_l
  Constant_x_l_d73c0 : Constant  Value=x_l
  Constant_x_l_ea8cc : Constant  Value=x_l
  Constant_x_qd_51b93 : Constant  Value=x_qd
  Constant_x_qd_6494e : Constant  Value=x_qd
  Constant_x_qd_7b45f : Constant  Value=x_qd
  Constant_x_qdd_04121 : Constant  Value=x_qdd
  Constant_x_qdd_7e2c0 : Constant  Value=x_qdd
  Constant_x_qdd_eecd9 : Constant  Value=x_qdd
  Divide_13fd6 : Product  Inputs=*/
  Divide_2609d : Product  Inputs=*/
  Divide_2c463 : Product  Inputs=*/
  Divide_44045 : Product  Inputs=*/
  Divide_78285 : Product  Inputs=*/
  Divide_da017 : Product  Inputs=*/
  Product_04892 : Product
  Product_0d825 : Product
  Product_11842 : Product
  Product_12f84 : Product
  Product_29da9 : Product
  Product_442b7 : Product
  Product_6ffd8 : Product
  Product_84eaa : Product
  Product_8855b : Product
  Product_a6848 : Product
  Product_acd52 : Product
  Subtract_2628b : Sum  Inputs=+-
  Subtract_2fb84 : Sum  Inputs=+-
  Subtract_32aa4 : Sum  Inputs=+-
  Subtract_5b0de : Sum  Inputs=+-
  Subtract_6e954 : Sum  Inputs=+-
  Subtract_a77ba : Sum  Inputs=+-
  Subtract_bbbd9 : Sum  Inputs=+-
  Blockout_T_e_SG_D_2_01d05 : Outport
  wires:
  Constant_-1_b2676/1 -> Product_29da9/1
  Divide_2609d/1 -> Subtract_a77ba/1
  Constant_-1_ef431/1 -> Product_11842/1
  Constant_x_l_d57ae/1 -> Product_11842/2
  Constant_x_qd_6494e/1 -> Subtract_6e954/1
  Product_acd52/1 -> Divide_2609d/1
  Product_11842/1 -> Add_1c286/1
  Divide_2c463/1 -> Subtract_2fb84/2
  Constant_x_qdd_7e2c0/1 -> Subtract_6e954/2
  Constant_x_qdd_04121/1 -> Divide_44045/2
  Constant_x_ddd_321b6/1 -> Subtract_32aa4/2
  Constant_x_qdd_eecd9/1 -> Add_1c286/2
  Constant_x_l_34d03/1 -> Product_29da9/2
  Constant_-1_0c5b4/1 -> Product_442b7/1
  Constant_x_l_b2fa4/1 -> Product_442b7/2
  Constant_-1_82549/1 -> Product_8855b/1
  State_psi_1d_SG_D_2_ae46f/1 -> Product_8855b/2
  Constant_x_dd_59712/1 -> Subtract_32aa4/1
  Divide_78285/1 -> Subtract_a77ba/2
  State_psi_gq_SG_D_2_e2d2d/1 -> Product_acd52/1
  Add_1c286/1 -> Product_acd52/2
  Subtract_a77ba/1 -> Add_8d046/1
  Constant_x_dd_02821/1 -> Subtract_bbbd9/1
  Product_29da9/1 -> Add_1b351/1
  Product_0d825/1 -> Product_84eaa/1
  Constant_x_qd_51b93/1 -> Add_1b351/2
  State_psi_kq_SG_D_2_b5b81/1 -> Product_a6848/1
  Subtract_6e954/1 -> Product_a6848/2
  Product_442b7/1 -> Add_e4b0b/1
  State_psi_q_SG_D_2_b8bd3/1 -> Product_6ffd8/1
  Constant_x_qd_7b45f/1 -> Add_e4b0b/2
  Product_8855b/1 -> Product_04892/1
  Divide_da017/1 -> Add_90198/2
  Subtract_32aa4/1 -> Product_04892/2
  Constant_x_l_d73c0/1 -> Subtract_bbbd9/2
  Constant_x_ddd_94546/1 -> Subtract_2628b/1
  Constant_x_dd_0cca3/1 -> Subtract_5b0de/1
  Constant_x_l_99a40/1 -> Subtract_2628b/2
  Add_90198/1 -> Blockout_T_e_SG_D_2_01d05/1
  Add_1b351/1 -> Divide_2609d/2
  Product_a6848/1 -> Divide_78285/1
  Product_84eaa/1 -> Divide_44045/1
  State_psi_d_SG_D_2_5c155/1 -> Product_0d825/2
  Add_e4b0b/1 -> Divide_78285/2
  Product_04892/1 -> Divide_13fd6/1
  Subtract_bbbd9/1 -> Divide_13fd6/2
  Constant_x_l_ea8cc/1 -> Subtract_5b0de/2
  State_psi_fd_SG_D_2_fdba3/1 -> Product_12f84/1
  Constant_x_ddd_b1f49/1 -> Divide_da017/2
  Product_6ffd8/1 -> Divide_da017/1
  Subtract_2628b/1 -> Product_12f84/2
  Divide_13fd6/1 -> Add_e613b/1
  State_psi_d_SG_D_2_c3c7e/1 -> Add_e613b/2
  Add_e613b/1 -> Subtract_2fb84/1
  Product_12f84/1 -> Divide_2c463/1
  Subtract_5b0de/1 -> Divide_2c463/2
  Constant_-1_84d88/1 -> Product_0d825/1
  State_psi_q_SG_D_2_2791a/1 -> Add_8d046/2
  Add_8d046/1 -> Product_84eaa/2
  Subtract_2fb84/1 -> Product_6ffd8/2
  Divide_44045/1 -> Add_90198/1

== system IEEE30_case/SG_D_2/d_E_fd_SG_D_2_block ==
  note: d_E_fd_SG_D_2 in IEEE30_case
      | $\frac{V_{f,\mathrm{SG},D,2}-E_{\mathrm{fd},\mathrm{SG},D,2}\,K_{E}}{T_{E}}$
      | Automatically generated on 2025-11-01 18:31:44 .
  State_E_fd_SG_D_2_d1f2e : Inport
  State_V_f_SG_D_2_b9fa9 : Inport  Port=2
  Add_11b50 : Sum
  Constant_-1_7954f : Constant  Value=-1
  Constant_K_E_d4951 : Constant  Value=K_E
  Constant_T_E_b3470 : Constant  Value=T_E
  Divide_db987 : Product  Inputs=*/
  Product_32b53 : Product
  Product_7df3a : Product
  Blockout_d_E_fd_SG_D_2_39068 : Outport
  wires:
  Constant_-1_7954f/1 -> Product_7df3a/1
  State_E_fd_SG_D_2_d1f2e/1 -> Product_7df3a/2
  Product_7df3a/1 -> Product_32b53/1
  Constant_K_E_d4951/1 -> Product_32b53/2
  Product_32b53/1 -> Add_11b50/1
  Constant_T_E_b3470/1 -> Divide_db987/2
  State_V_f_SG_D_2_b9fa9/1 -> Add_11b50/2
  Add_11b50/1 -> Divide_db987/1
  Divide_db987/1 -> Blockout_d_E_fd_SG_D_2_39068/1

== system IEEE30_case/SG_D_2/d_Px_1_SG_D_2_block ==
  note: d_Px_1_SG_D_2 in IEEE30_case
      | $\frac{w_{\mathrm{SG},D,2}-2\,\pi \,f_{0}}{T_{w}}-\frac{\mathrm{Px}_{1,\mathrm{SG},D,2}}{T_{w}}$
      | Automatically generated on 2025-11-01 18:31:45 .
  State_Px_1_SG_D_2_b4144 : Inport
  State_w_SG_D_2_0d596 : Inport  Port=2
  Add_89ca7 : Sum
  Add_bef6e : Sum
  Constant_-1_8b12b : Constant  Value=-1
  Constant_-2.0_94173 : Constant  Value=-2.0
  Constant_T_w_023b7 : Constant  Value=T_w
  Constant_T_w_a2273 : Constant  Value=T_w
  Constant_f0_62502 : Constant  Value=f0
  Constant_pi_32f0e : Constant  Value=pi
  Divide_5186e : Product  Inputs=*/
  Divide_be575 : Product  Inputs=*/
  Product_031b7 : Product
  Product_07a56 : Product
  Product_79daf : Product
  Blockout_d_Px_1_SG_D_2_215fb : Outport
  wires:
  Constant_-2.0_94173/1 -> Product_031b7/1
  State_w_SG_D_2_0d596/1 -> Add_89ca7/2
  Constant_pi_32f0e/1 -> Product_031b7/2
  Product_031b7/1 -> Product_79daf/1
  Constant_f0_62502/1 -> Product_79daf/2
  Constant_-1_8b12b/1 -> Product_07a56/1
  State_Px_1_SG_D_2_b4144/1 -> Product_07a56/2
  Product_79daf/1 -> Add_89ca7/1
  Product_07a56/1 -> Divide_be575/1
  Constant_T_w_a2273/1 -> Divide_be575/2
  Add_89ca7/1 -> Divide_5186e/1
  Constant_T_w_023b7/1 -> Divide_5186e/2
  Divide_be575/1 -> Add_bef6e/1
  Divide_5186e/1 -> Add_bef6e/2
  Add_bef6e/1 -> Blockout_d_Px_1_SG_D_2_215fb/1

== system IEEE30_case/SG_D_2/d_Px_2_SG_D_2_block ==
  note: d_Px_2_SG_D_2 in IEEE30_case
      | $\frac{\mathrm{Px}_{1,\mathrm{SG},D,2}-T_{2}\,\left(\frac{\mathrm{Px}_{1,\mathrm{SG},D,2}}{T_{w}}-\frac{w_{\mathrm{SG},D,2}-2\,\pi \,f_{0}}{T_{w}}\right)}{T_{1}}-\frac{\mathrm{Px}_{2,\mathrm{SG},D,2}}{T_{1}}$
      | Automatically generated on 2025-11-01 18:31:47 .
  State_Px_2_SG_D_2_06380 : Inport
  State_Px_1_SG_D_2_4e32d : Inport  Port=2
  State_Px_1_SG_D_2_8c524 : Inport  Port=3
  State_w_SG_D_2_2a02e : Inport  Port=4
  Add_290b2 : Sum
  Add_2d06c : Sum
  Add_a0c0b : Sum
  Add_b0973 : Sum
  Constant_-1_0e587 : Constant  Value=-1
  Constant_-1_5fa0f : Constant  Value=-1
  Constant_-2.0_be430 : Constant  Value=-2.0
  Constant_T_1_c8f26 : Constant  Value=T_1
  Constant_T_1_fb541 : Constant  Value=T_1
  Constant_T_2_e907b : Constant  Value=T_2
  Constant_T_w_3c60f : Constant  Value=T_w
  Constant_T_w_4296b : Constant  Value=T_w
  Constant_f0_589cb : Constant  Value=f0
  Constant_pi_f13d7 : Constant  Value=pi
  Divide_28183 : Product  Inputs=*/
  Divide_61d17 : Product  Inputs=*/
  Divide_a172d : Product  Inputs=*/
  Divide_b8671 : Product  Inputs=*/
  Product_23a66 : Product
  Product_3248d : Product
  Product_3a904 : Product
  Product_8efd7 : Product
  Product_cf4e4 : Product
  Blockout_d_Px_2_SG_D_2_fe4d9 : Outport
  wires:
  Constant_-1_0e587/1 -> Product_3a904/1
  Constant_-2.0_be430/1 -> Product_cf4e4/1
  Product_23a66/1 -> Add_2d06c/2
  State_w_SG_D_2_2a02e/1 -> Add_a0c0b/2
  Constant_pi_f13d7/1 -> Product_cf4e4/2
  Product_cf4e4/1 -> Product_8efd7/1
  State_Px_1_SG_D_2_8c524/1 -> Product_3248d/2
  Constant_f0_589cb/1 -> Product_8efd7/2
  State_Px_2_SG_D_2_06380/1 -> Product_3a904/2
  Constant_-1_5fa0f/1 -> Product_3248d/1
  Product_8efd7/1 -> Add_a0c0b/1
  Product_3248d/1 -> Divide_a172d/1
  Constant_T_w_4296b/1 -> Divide_a172d/2
  Add_a0c0b/1 -> Divide_61d17/1
  Constant_T_w_3c60f/1 -> Divide_61d17/2
  Divide_a172d/1 -> Add_290b2/1
  Divide_61d17/1 -> Add_290b2/2
  Constant_T_2_e907b/1 -> Product_23a66/1
  Add_290b2/1 -> Product_23a66/2
  State_Px_1_SG_D_2_4e32d/1 -> Add_2d06c/1
  Product_3a904/1 -> Divide_28183/1
  Constant_T_1_c8f26/1 -> Divide_28183/2
  Add_2d06c/1 -> Divide_b8671/1
  Constant_T_1_fb541/1 -> Divide_b8671/2
  Divide_28183/1 -> Add_b0973/1
  Divide_b8671/1 -> Add_b0973/2
  Add_b0973/1 -> Blockout_d_Px_2_SG_D_2_fe4d9/1

== system IEEE30_case/SG_D_2/d_Px_3_SG_D_2_block ==
  note: d_Px_3_SG_D_2 in IEEE30_case
      | $\frac{\mathrm{Px}_{2,\mathrm{SG},D,2}+T_{4}\,\left(\frac{\mathrm{Px}_{1,\mathrm{SG},D,2}-T_{2}\,\left(\frac{\mathrm{Px}_{1,\mathrm{SG},D,2}}{T_{w}}-\frac{w_{\mathrm{SG},D,2}-2\,\pi \,f_{0}}{T_{w}}\right)}{T_{1}}-\frac{\mathrm{Px}_{2,\mathrm{SG},D,2}}{T_{1}}\right)}{T_{3}}-\frac{\mathrm{Px}_{3,\mathrm{SG},D,2}}{T_{3}}$
      | Automatically generated on 2025-11-01 18:31:49 .
  State_Px_3_SG_D_2_dac62 : Inport
  State_Px_2_SG_D_2_f8442 : Inport  Port=2
  State_Px_2_SG_D_2_0d955 : Inport  Port=3
  State_Px_1_SG_D_2_7331f : Inport  Port=4
  State_Px_1_SG_D_2_9d5b2 : Inport  Port=5
  State_w_SG_D_2_59107 : Inport  Port=6
  Add_3d1f4 : Sum
  Add_60d48 : Sum
  Add_7530a : Sum
  Add_84208 : Sum
  Add_c8064 : Sum
  Add_cd79f : Sum
  Constant_-1_03ded : Constant  Value=-1
  Constant_-1_1fdf0 : Constant  Value=-1
  Constant_-1_d5c97 : Constant  Value=-1
  Constant_-2.0_06b55 : Constant  Value=-2.0
  Constant_T_1_2fa27 : Constant  Value=T_1
  Constant_T_1_58779 : Constant  Value=T_1
  Constant_T_2_7bc1b : Constant  Value=T_2
  Constant_T_3_e830c : Constant  Value=T_3
  Constant_T_3_f24dd : Constant  Value=T_3
  Constant_T_4_7a18c : Constant  Value=T_4
  Constant_T_w_01570 : Constant  Value=T_w
  Constant_T_w_7c2ee : Constant  Value=T_w
  Constant_f0_64012 : Constant  Value=f0
  Constant_pi_d1391 : Constant  Value=pi
  Divide_02d6a : Product  Inputs=*/
  Divide_7fcaa : Product  Inputs=*/
  Divide_9dac1 : Product  Inputs=*/
  Divide_c57c9 : Product  Inputs=*/
  Divide_c8514 : Product  Inputs=*/
  Divide_ff391 : Product  Inputs=*/
  Product_50271 : Product
  Product_682d1 : Product
  Product_81496 : Product
  Product_a741c : Product
  Product_ce939 : Product
  Product_fc9b0 : Product
  Product_fe667 : Product
  Blockout_d_Px_3_SG_D_2_f118f : Outport
  wires:
  Constant_-2.0_06b55/1 -> Product_a741c/1
  State_w_SG_D_2_59107/1 -> Add_84208/2
  Add_cd79f/1 -> Divide_7fcaa/1
  Constant_pi_d1391/1 -> Product_a741c/2
  Constant_-1_d5c97/1 -> Product_fc9b0/1
  Product_a741c/1 -> Product_fe667/1
  State_Px_2_SG_D_2_0d955/1 -> Product_fc9b0/2
  State_Px_1_SG_D_2_9d5b2/1 -> Product_682d1/2
  Divide_7fcaa/1 -> Add_c8064/2
  Constant_f0_64012/1 -> Product_fe667/2
  Constant_-1_03ded/1 -> Product_682d1/1
  Product_fe667/1 -> Add_84208/1
  Product_682d1/1 -> Divide_c8514/1
  Constant_T_w_7c2ee/1 -> Divide_c8514/2
  Divide_c57c9/1 -> Add_c8064/1
  Add_84208/1 -> Divide_02d6a/1
  Product_ce939/1 -> Add_3d1f4/2
  Constant_T_w_01570/1 -> Divide_02d6a/2
  Divide_c8514/1 -> Add_60d48/1
  State_Px_1_SG_D_2_7331f/1 -> Add_3d1f4/1
  Divide_02d6a/1 -> Add_60d48/2
  Constant_-1_1fdf0/1 -> Product_81496/1
  Constant_T_2_7bc1b/1 -> Product_ce939/1
  Add_60d48/1 -> Product_ce939/2
  Product_fc9b0/1 -> Divide_ff391/1
  Constant_T_1_2fa27/1 -> Divide_ff391/2
  Add_3d1f4/1 -> Divide_9dac1/1
  Constant_T_1_58779/1 -> Divide_9dac1/2
  Divide_ff391/1 -> Add_7530a/1
  Divide_9dac1/1 -> Add_7530a/2
  Constant_T_4_7a18c/1 -> Product_50271/1
  Add_7530a/1 -> Product_50271/2
  State_Px_3_SG_D_2_dac62/1 -> Product_81496/2
  State_Px_2_SG_D_2_f8442/1 -> Add_cd79f/1
  Product_50271/1 -> Add_cd79f/2
  Product_81496/1 -> Divide_c57c9/1
  Constant_T_3_e830c/1 -> Divide_c57c9/2
  Constant_T_3_f24dd/1 -> Divide_7fcaa/2
  Add_c8064/1 -> Blockout_d_Px_3_SG_D_2_f118f/1

== system IEEE30_case/SG_D_2/d_R_f_SG_D_2_block ==
  note: d_R_f_SG_D_2 in IEEE30_case
      | $-\frac{R_{f,\mathrm{SG},D,2}-\frac{E_{\mathrm{fd},\mathrm{SG},D,2}\,K_{F}}{T_{F}}}{T_{F}}$
      | Automatically generated on 2025-11-01 18:31:43 .
  State_E_fd_SG_D_2_d5c8d : Inport
  State_R_f_SG_D_2_6571e : Inport  Port=2
  Constant_K_F_17094 : Constant  Value=K_F
  Constant_T_F_b1a0c : Constant  Value=T_F
  Constant_T_F_b7863 : Constant  Value=T_F
  Divide_80a77 : Product  Inputs=*/
  Divide_8ce88 : Product  Inputs=*/
  Product_9d4f7 : Product
  Subtract_31629 : Sum  Inputs=+-
  Blockout_d_R_f_SG_D_2_b95c5 : Outport
  wires:
  Constant_T_F_b7863/1 -> Divide_8ce88/2
  State_E_fd_SG_D_2_d5c8d/1 -> Product_9d4f7/1
  Constant_K_F_17094/1 -> Product_9d4f7/2
  State_R_f_SG_D_2_6571e/1 -> Subtract_31629/2
  Product_9d4f7/1 -> Divide_8ce88/1
  Divide_8ce88/1 -> Subtract_31629/1
  Constant_T_F_b1a0c/1 -> Divide_80a77/2
  Subtract_31629/1 -> Divide_80a77/1
  Divide_80a77/1 -> Blockout_d_R_f_SG_D_2_b95c5/1

== system IEEE30_case/SG_D_2/d_T_m_SG_D_2_block ==
  note: d_T_m_SG_D_2 in IEEE30_case
      | $-\frac{T_{m,\mathrm{SG},D,2}-T_{0}+\frac{\mathrm{SpeedPara}\,\left(w_{\mathrm{SG},D,2}-w_{\mathrm{ref}}\right)}{2\,f_{0}\,\pi }}{T_{\mathrm{speed}}}$
      | Automatically generated on 2025-11-01 18:31:34 .
  State_w_SG_D_2_b536b : Inport
  State_T_m_SG_D_2_c8c02 : Inport  Port=2
  Add_b7907 : Sum
  Add_f543b : Sum
  Constant_-1_4929f : Constant  Value=-1
  Constant_2.0_3f1fe : Constant  Value=2.0
  Constant_SpeedPara_2ef9d : Constant  Value=SpeedPara
  Constant_T_0_a357a : Constant  Value=T_0
  Constant_T_speed_af8fd : Constant  Value=T_speed
  Constant_f0_a764a : Constant  Value=f0
  Constant_pi_00277 : Constant  Value=pi
  Constant_w_ref_9a0fd : Constant  Value=w_ref
  Divide_4b494 : Product  Inputs=*/
  Divide_b64ff : Product  Inputs=*/
  Product_291a8 : Product
  Product_d8093 : Product
  Product_e2fe2 : Product
  Product_f0253 : Product
  Subtract_f1eaa : Sum  Inputs=+-
  Blockout_d_T_m_SG_D_2_a9295 : Outport
  wires:
  Constant_pi_00277/1 -> Product_e2fe2/2
  Constant_-1_4929f/1 -> Product_d8093/1
  Constant_w_ref_9a0fd/1 -> Add_b7907/2
  State_w_SG_D_2_b536b/1 -> Product_d8093/2
  Product_d8093/1 -> Add_b7907/1
  Add_f543b/1 -> Subtract_f1eaa/1
  Add_b7907/1 -> Product_f0253/2
  Constant_2.0_3f1fe/1 -> Product_e2fe2/1
  Constant_SpeedPara_2ef9d/1 -> Product_f0253/1
  Product_e2fe2/1 -> Product_291a8/1
  Constant_f0_a764a/1 -> Product_291a8/2
  Product_f0253/1 -> Divide_b64ff/1
  Product_291a8/1 -> Divide_b64ff/2
  Divide_b64ff/1 -> Add_f543b/1
  Constant_T_0_a357a/1 -> Add_f543b/2
  State_T_m_SG_D_2_c8c02/1 -> Subtract_f1eaa/2
  Subtract_f1eaa/1 -> Divide_4b494/1
  Constant_T_speed_af8fd/1 -> Divide_4b494/2
  Divide_4b494/1 -> Blockout_d_T_m_SG_D_2_a9295/1
